simulink library "Springs_Independent"  (R2018b)
settings: Solver=VariableStepAuto  StartTime=0.0  StopTime=10.0  RelTol=1e-3
libraries: fl_lib x6, sm_car_lib x6
Description:
  | Component of Simscape Vehicle Templates Library
  | 
  | Copyright 2018-2020 The MathWorks, Inc.
settings Model: Creator=smiller  LastModifiedBy=smiller

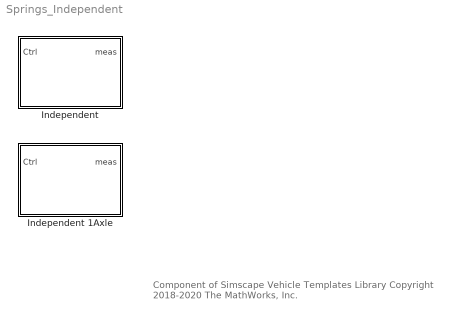
== system Springs_Independent ==
  note: Component of Simscape Vehicle Templates Library
      | Copyright 2018-2020 The MathWorks, Inc.
  Independent : Subsystem  VariantControl=Independent  mask(Independent Springs){InitTriggerDropdown=0}
      mask prompts: InitTriggerDropdown "Initialization Trigger Dropdown"
      mask help: Springs with no physical connections to one another.
      mask init:
      | curblk = gcb;
      | 
      | % Trigger Mask Initialization for 
      | % variant subsystems below this level
      | sm_car_lib_maskInitTrigger(curblk);
      mask TypeOptions InitTriggerDropdown: 0 | 1
  Independent 1Axle : Subsystem  VariantControl=Independent  mask(Independent Springs){InitTriggerDropdown=0}
      mask prompts: InitTriggerDropdown "Initialization Trigger Dropdown"
      mask help: Springs with no physical connections to one another.
      mask init:
      | curblk = gcb;
      | 
      | % Trigger Mask Initialization for 
      | % variant subsystems below this level
      | sm_car_lib_maskInitTrigger(curblk);
      mask TypeOptions InitTriggerDropdown: 0 | 1

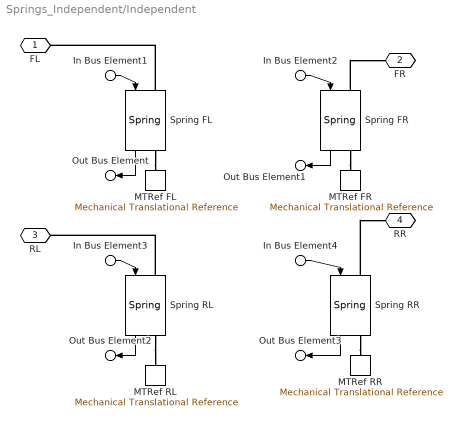
== system Springs_Independent/Independent ==
  In Bus Element1 : Inport  PortName=Ctrl  Element=FL
  In Bus Element2 : Inport  PortName=Ctrl  Element=FR
  In Bus Element3 : Inport  PortName=Ctrl  Element=RL
  In Bus Element4 : Inport  PortName=Ctrl  Element=RR
  MTRef FL : fl_lib/Mechanical/Translational Elements/Mechanical Translational Reference
  MTRef FR : fl_lib/Mechanical/Translational Elements/Mechanical Translational Reference
  MTRef RL : fl_lib/Mechanical/Translational Elements/Mechanical Translational Reference
  MTRef RR : fl_lib/Mechanical/Translational Elements/Mechanical Translational Reference
  Spring FL : sm_car_lib/Springs Dampers/Spring  VariantControl=Variant1  Spring=Spring.Front  VariantLabel=Spring.Front.class.Value  InitTriggerDropdown=0
      settings: AttributesFormatString=%<ActiveVariant>
  Spring FR : sm_car_lib/Springs Dampers/Spring  VariantControl=Variant1  Spring=Spring.Front  VariantLabel=Spring.Front.class.Value  InitTriggerDropdown=0
      settings: AttributesFormatString=%<ActiveVariant>
  Spring RL : sm_car_lib/Springs Dampers/Spring  VariantControl=Variant1  Spring=Spring.Rear  VariantLabel=Spring.Rear.class.Value  InitTriggerDropdown=0
      settings: AttributesFormatString=%<ActiveVariant>
  Spring RR : sm_car_lib/Springs Dampers/Spring  VariantControl=Variant1  Spring=Spring.Rear  VariantLabel=Spring.Rear.class.Value  InitTriggerDropdown=0
      settings: AttributesFormatString=%<ActiveVariant>
  FL : PMIOPort  Side=Left
  FR : PMIOPort  Port=2  Side=Right
  RL : PMIOPort  Port=3  Side=Left
  RR : PMIOPort  Port=4  Side=Right
  Out Bus Element : Outport  PortName=meas  Element=FL
  Out Bus Element1 : Outport  PortName=meas  Element=FR
  Out Bus Element2 : Outport  PortName=meas  Element=RL
  Out Bus Element3 : Outport  PortName=meas  Element=RR
  wires:
  Spring RR/1 -> Out Bus Element3/1
  In Bus Element4/1 -> Spring RR/1
  Spring RL/1 -> Out Bus Element2/1
  In Bus Element3/1 -> Spring RL/1
  Spring FR/1 -> Out Bus Element1/1
  In Bus Element2/1 -> Spring FR/1
  Spring FL/1 -> Out Bus Element/1
  In Bus Element1/1 -> Spring FL/1
  connections:
  Spring FL/RConn1 -- MTRef FL/LConn1
  Spring FL/LConn1 -- FL/RConn1
  Spring RL/RConn1 -- MTRef RL/LConn1
  Spring RL/LConn1 -- RL/RConn1
  Spring RR/RConn1 -- MTRef RR/LConn1
  Spring RR/LConn1 -- RR/RConn1
  Spring FR/RConn1 -- MTRef FR/LConn1
  Spring FR/LConn1 -- FR/RConn1

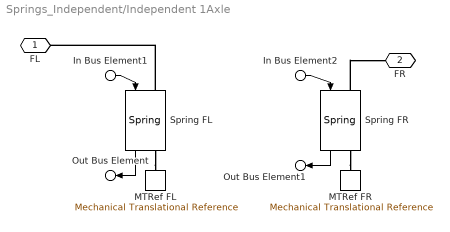
== system Springs_Independent/Independent 1Axle ==
  In Bus Element1 : Inport  PortName=Ctrl  Element=FL
  In Bus Element2 : Inport  PortName=Ctrl  Element=FR
  MTRef FL : fl_lib/Mechanical/Translational Elements/Mechanical Translational Reference
  MTRef FR : fl_lib/Mechanical/Translational Elements/Mechanical Translational Reference
  Spring FL : sm_car_lib/Springs Dampers/Spring  VariantControl=Variant1  Spring=Spring.Front  VariantLabel=Spring.Front.class.Value  InitTriggerDropdown=0
      settings: AttributesFormatString=%<ActiveVariant>
  Spring FR : sm_car_lib/Springs Dampers/Spring  VariantControl=Variant1  Spring=Spring.Front  VariantLabel=Spring.Front.class.Value  InitTriggerDropdown=0
      settings: AttributesFormatString=%<ActiveVariant>
  FL : PMIOPort  Side=Left
  FR : PMIOPort  Port=2  Side=Right
  Out Bus Element : Outport  PortName=meas  Element=FL
  Out Bus Element1 : Outport  PortName=meas  Element=FR
  wires:
  In Bus Element1/1 -> Spring FL/1
  Spring FL/1 -> Out Bus Element/1
  In Bus Element2/1 -> Spring FR/1
  Spring FR/1 -> Out Bus Element1/1
  connections:
  Spring FR/LConn1 -- FR/RConn1
  Spring FR/RConn1 -- MTRef FR/LConn1
  Spring FL/LConn1 -- FL/RConn1
  Spring FL/RConn1 -- MTRef FL/LConn1
